simulink model "BICYCLE"  (R2022b)
settings: Solver=VariableStepAuto  StartTime=0.0  StopTime=10.0  RelTol=1e-3
settings Model: Creator=박재두  LastModifiedBy=박재두
settings DataIOCC: ExternalInput=[T', SPD']  LoadExternalInput=on  SaveFormat=Array

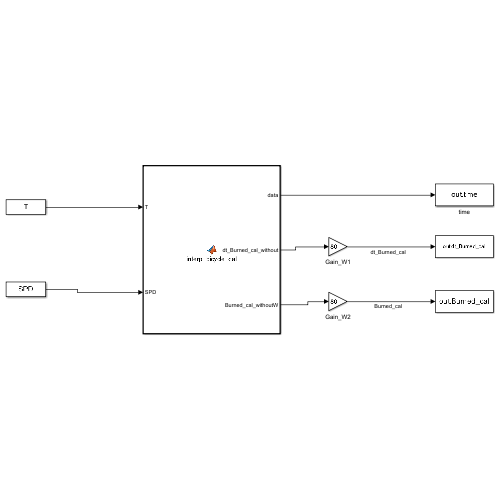
[thumbnail: Simulink's stored preview of the top-level diagram]
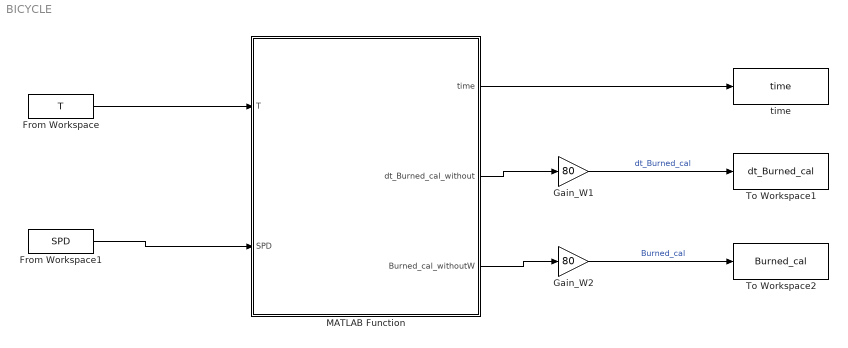
== system BICYCLE ==
  From Workspace : FromWorkspace  VariableName=T
  From Workspace1 : FromWorkspace  VariableName=SPD
  Gain_W1 : Gain  Gain=80
  Gain_W2 : Gain  Gain=80
  MATLAB Function : MATLAB Function  TreatAsAtomicUnit=on
  To Workspace1 : ToWorkspace  VariableName=dt_Burned_cal  SampleTime=-1
  To Workspace2 : ToWorkspace  VariableName=Burned_cal  SampleTime=-1
  time : ToWorkspace  VariableName=time  SampleTime=-1
  wires:
  From Workspace1/1 -> MATLAB Function/2(SPD)
  From Workspace/1 -> MATLAB Function/1(T)
  MATLAB Function/2(dt_Burned_cal_without) -> Gain_W1/1
  MATLAB Function/3(Burned_cal_withoutW) -> Gain_W2/1
  Gain_W1/1 -> To Workspace1/1  "dt_Burned_cal"
  Gain_W2/1 -> To Workspace2/1  "Burned_cal"
  MATLAB Function/1(time) -> time/1

== matlab function BICYCLE/MATLAB Function ==
  data: time output; T input; SPD input; dt_Burned_cal_without output; Burned_cal_withoutW output
function [time, dt_Burned_cal_without, Burned_cal_withoutW] = interp_bicycle_cal(T, SPD)
% [time,dt_Burned_cal,Burned_cal] = interp_bicycle_cal_matonly(Time,speed,Body Wegiht)
% Burned_cal(행백터): 누적된 칼로리 소모량
% dt_Burned_cal(행벡터): 순간 칼로리 소모량
% 21013292 박재두

% Burned_cal : 총 소모된 칼로리(벡터)
% T(sec) : 측정 후 지난 시간(벡터)
% SPD(km) : 측정 시각의 속도(벡터)
% W(kg) : 몸무게(스칼라)

SPD = SPD(2,:); % 시간에 대한 source, 2행으로 받아온 source를 행벡터로 만들기
T = T(2,:);

% 보간법 사용
new_t = 1:1:T(end);
time = new_t;
new_speed = interp1(T, SPD, new_t);

% MET : Metabolic Equivalent of Task (MET)
dt_Burned_cal_without = zeros(1, length(new_speed));
Burned_cal_withoutW = zeros(1, length(new_speed));
burned_cal_withoutW = 0;

for i = 2:length(new_speed)
    spd = new_speed(i);
    if spd>=30
        met = 9; 
    elseif spd>=20
        met = 8;         
    elseif spd>=16
        met = 5;   
    elseif spd>=12
        met = 4;
    elseif spd>=8
        met = 3;
    elseif spd>=4
        met = 2.5;
    elseif spd>=2
        met = 2;
    else
        met = 1.0;
    end

    dt_burned_cal_withoutW = met*(new_t(i) - new_t(i-1))*(1/60)*(1/60);
    dt_Burned_cal_without(i) = dt_burned_cal_withoutW;
    burned_cal_withoutW = burned_cal_withoutW + dt_burned_cal_withoutW;
    Burned_cal_withoutW(i) = burned_cal_withoutW;
end
% time,dt_Burned_cal_without,Burned_cal_withoutW은 행벡터
% 벡터를 2행 크기의 행렬로 만드는 중
dt_Burned_cal_without = [time;dt_Burned_cal_without];
Burned_cal_withoutW = [time;Burned_cal_withoutW];
end
